simulink model "gm_FCS_MPC_3Phase_SPMSM_TEST1"  (R2022a)
settings: Solver=ode23t  StartTime=0.0  StopTime=0.2  RelTol=1e-3  AbsTol=1e-3  EnableMultiTasking=on
undefined symbols (not defined in the file or in its folder): f_c, Ld, Lq, np, psiPM, R, T_50MHz, u_dc
libraries: dspsigops x31, hdlmdlgenlib x28, ee_lib x22, nesl_utility x22, fl_lib x21, simulink x7
(part 3 of 5)

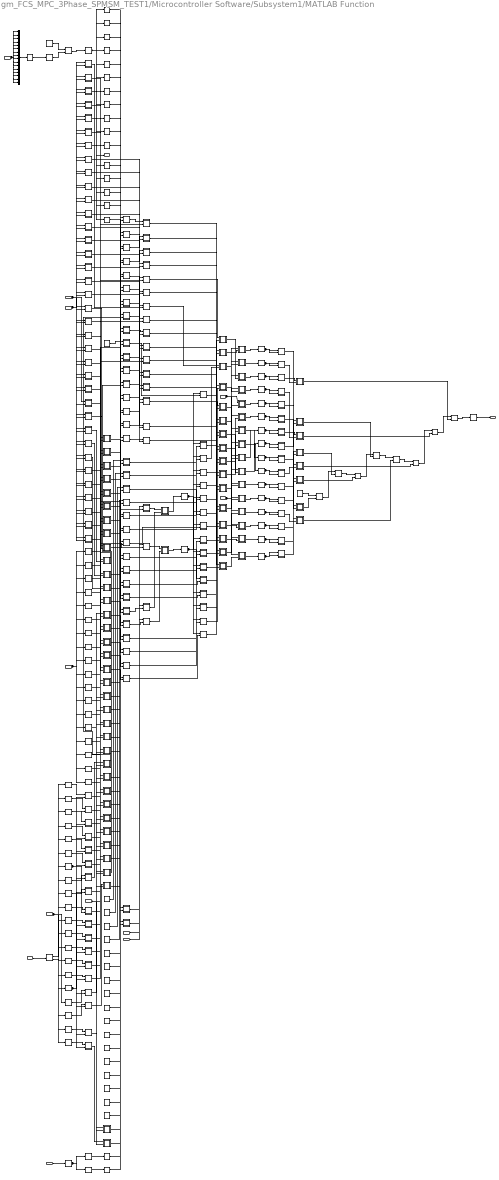
== system gm_FCS_MPC_3Phase_SPMSM_TEST1/Microcontroller Software/Subsystem1/MATLAB Function ==
  u_dc_link : Inport  OutDataTypeStr=single  PortDimensions=1  SampleTime=1e-10
  i_ph_ctrl_alpha : Inport  Port=2  OutDataTypeStr=single  PortDimensions=1  SampleTime=1e-10
  i_ph_ctrl_beta : Inport  Port=3  OutDataTypeStr=single  PortDimensions=1  SampleTime=1e-10
  omega_el : Inport  Port=4  OutDataTypeStr=single  PortDimensions=1  SampleTime=1e-10
  theta_el : Inport  Port=5  OutDataTypeStr=single  PortDimensions=1  SampleTime=1e-10
  Rs : Inport  Port=6  OutDataTypeStr=single  PortDimensions=1  SampleTime=1e-10
  reciprocal_Ls : Inport  Port=7  OutDataTypeStr=single  PortDimensions=1  SampleTime=1e-10
  psiPM : Inport  Port=8  OutDataTypeStr=single  PortDimensions=1  SampleTime=1e-10
  ialpha_ref : Inport  Port=9  OutDataTypeStr=single  PortDimensions=1  SampleTime=1e-10
  ibeta_ref : Inport  Port=10  OutDataTypeStr=single  PortDimensions=1  SampleTime=1e-10
  SampleTime : Inport  Port=11  OutDataTypeStr=single  PortDimensions=1  SampleTime=1e-10
  vk : Inport  Port=12  OutDataTypeStr=single  PortDimensions=[2]  SampleTime=1e-10
  Assignment : Assignment  SampleTime=1e-10  IndexOptions=Index vector (dialog)  Indices=double(8)  OutputSizes=double(0)
  Assignment1 : Assignment  SampleTime=1e-10  IndexOptions=Index vector (dialog)  Indices=double(7)  OutputSizes=double(0)
  Assignment2 : Assignment  SampleTime=1e-10  IndexOptions=Index vector (dialog)  Indices=double(6)  OutputSizes=double(0)
  Assignment3 : Assignment  SampleTime=1e-10  IndexOptions=Index vector (dialog)  Indices=double(5)  OutputSizes=double(0)
  Assignment4 : Assignment  SampleTime=1e-10  IndexOptions=Index vector (dialog)  Indices=double(4)  OutputSizes=double(0)
  Assignment5 : Assignment  SampleTime=1e-10  IndexOptions=Index vector (dialog)  Indices=double(3)  OutputSizes=double(0)
  Assignment6 : Assignment  SampleTime=1e-10  IndexOptions=Index vector (dialog)  Indices=double(2)  OutputSizes=double(0)
  Assignment7 : Assignment  SampleTime=1e-10  IndexOptions=Index vector (dialog)  Indices=double(1)  OutputSizes=double(0)
  Reshape : Reshape
  Reshape1 : Reshape  OutputDimensionality=Column vector (2-D)
  Selector : Selector  NumberOfDimensions=2  SampleTime=1e-10  IndexOptions=Index vector (dialog),Index vector (dialog)  Indices=double(2),double(8)  OutputSizes=double(0),double(0)
  Selector1 : Selector  NumberOfDimensions=2  SampleTime=1e-10  IndexOptions=Index vector (dialog),Index vector (dialog)  Indices=double(1),double(8)  OutputSizes=double(0),double(0)
  Selector10 : Selector  NumberOfDimensions=2  SampleTime=1e-10  IndexOptions=Index vector (dialog),Index vector (dialog)  Indices=double(2),double(4)  OutputSizes=double(0),double(0)
  Selector11 : Selector  NumberOfDimensions=2  SampleTime=1e-10  IndexOptions=Index vector (dialog),Index vector (dialog)  Indices=double(1),double(4)  OutputSizes=double(0),double(0)
  Selector12 : Selector  NumberOfDimensions=2  SampleTime=1e-10  IndexOptions=Index vector (dialog),Index vector (dialog)  Indices=double(2),double(3)  OutputSizes=double(0),double(0)
  Selector13 : Selector  NumberOfDimensions=2  SampleTime=1e-10  IndexOptions=Index vector (dialog),Index vector (dialog)  Indices=double(1),double(3)  OutputSizes=double(0),double(0)
  Selector14 : Selector  NumberOfDimensions=2  SampleTime=1e-10  IndexOptions=Index vector (dialog),Index vector (dialog)  Indices=double(2),double(2)  OutputSizes=double(0),double(0)
  Selector15 : Selector  NumberOfDimensions=2  SampleTime=1e-10  IndexOptions=Index vector (dialog),Index vector (dialog)  Indices=double(1),double(2)  OutputSizes=double(0),double(0)
  Selector16 : Selector  NumberOfDimensions=2  SampleTime=1e-10  IndexOptions=Index vector (dialog),Index vector (dialog)  Indices=double(2),double(1)  OutputSizes=double(0),double(0)
  Selector17 : Selector  NumberOfDimensions=2  SampleTime=1e-10  IndexOptions=Index vector (dialog),Index vector (dialog)  Indices=double(1),double(1)  OutputSizes=double(0),double(0)
  Selector2 : Selector  NumberOfDimensions=2  SampleTime=1e-10  IndexOptions=Index vector (dialog),Index vector (dialog)  Indices=double(2),double(7)  OutputSizes=double(0),double(0)
  Selector3 : Selector  NumberOfDimensions=2  SampleTime=1e-10  IndexOptions=Index vector (dialog),Index vector (dialog)  Indices=double(1),double(7)  OutputSizes=double(0),double(0)
  Selector4 : Selector  SampleTime=1e-10  IndexOptions=Index vector (dialog)  Indices=double(2)  OutputSizes=double(0)
  Selector5 : Selector  SampleTime=1e-10  IndexOptions=Index vector (dialog)  Indices=double(1)  OutputSizes=double(0)
  Selector6 : Selector  NumberOfDimensions=2  SampleTime=1e-10  IndexOptions=Index vector (dialog),Index vector (dialog)  Indices=double(2),double(6)  OutputSizes=double(0),double(0)
  Selector7 : Selector  NumberOfDimensions=2  SampleTime=1e-10  IndexOptions=Index vector (dialog),Index vector (dialog)  Indices=double(1),double(6)  OutputSizes=double(0),double(0)
  Selector8 : Selector  NumberOfDimensions=2  SampleTime=1e-10  IndexOptions=Index vector (dialog),Index vector (dialog)  Indices=double(2),double(5)  OutputSizes=double(0),double(0)
  Selector9 : Selector  NumberOfDimensions=2  SampleTime=1e-10  IndexOptions=Index vector (dialog),Index vector (dialog)  Indices=double(1),double(5)  OutputSizes=double(0),double(0)
  adder : Subsystem
      mask Display: disp('NFP\nadd');
  adder1 : Subsystem
      mask Display: disp('NFP\nadd');
  adder10 : Subsystem
      mask Display: disp('NFP\nadd');
  adder11 : Subsystem
      mask Display: disp('NFP\nadd');
  adder12 : Subsystem
      mask Display: disp('NFP\nadd');
  adder13 : Subsystem
      mask Display: disp('NFP\nadd');
  adder14 : Subsystem
      mask Display: disp('NFP\nadd');
  adder15 : Subsystem
      mask Display: disp('NFP\nadd');
  adder16 : Subsystem
      mask Display: disp('NFP\nadd');
  adder17 : Subsystem
      mask Display: disp('NFP\nadd');
  adder18 : Subsystem
      mask Display: disp('NFP\nadd');
  adder19 : Subsystem
      mask Display: disp('NFP\nadd');
  adder2 : Subsystem
      mask Display: disp('NFP\nadd');
  adder20 : Subsystem
      mask Display: disp('NFP\nadd');
  adder21 : Subsystem
      mask Display: disp('NFP\nadd');
  adder22 : Subsystem
      mask Display: disp('NFP\nadd');
  adder23 : Subsystem
      mask Display: disp('NFP\nadd');
  adder24 : Subsystem
      mask Display: disp('NFP\nadd');
  adder25 : Subsystem
      mask Display: disp('NFP\nadd');
  adder26 : Subsystem
      mask Display: disp('NFP\nadd');
  adder27 : Subsystem
      mask Display: disp('NFP\nadd');
  adder28 : Subsystem
      mask Display: disp('NFP\nadd');
  adder29 : Subsystem
      mask Display: disp('NFP\nadd');
  adder3 : Subsystem
      mask Display: disp('NFP\nadd');
  adder30 : Subsystem
      mask Display: disp('NFP\nadd');
  adder31 : Subsystem
      mask Display: disp('NFP\nadd');
  adder32 : Subsystem
      mask Display: disp('NFP\nadd');
  adder33 : Subsystem
      mask Display: disp('NFP\nadd');
  adder34 : Subsystem
      mask Display: disp('NFP\nadd');
  adder4 : Subsystem
      mask Display: disp('NFP\nadd');
  adder5 : Subsystem
      mask Display: disp('NFP\nadd');
  adder6 : Subsystem
      mask Display: disp('NFP\nadd');
  adder7 : Subsystem
      mask Display: disp('NFP\nadd');
  adder8 : Subsystem
      mask Display: disp('NFP\nadd');
  adder9 : Subsystem
      mask Display: disp('NFP\nadd');
  adder_outbuff : hdlmdlgenlib/Buffer
      settings: SourceProductBaseCode=SL
  adder_outbuff1 : hdlmdlgenlib/Buffer
      settings: SourceProductBaseCode=SL
  concatenate : Concatenate  NumInputs=16
  const{,1..3,5..18} (18 alike) : Constant  Value=single(1)  VectorParams1D=off  OutDataTypeStr=single  SampleTime=1e-10
  const4 : Constant  Value="repmat(single(0),[8  1])"  VectorParams1D=off  OutDataTypeStr=single  SampleTime=1e-10
  cos_to_sincos : Subsystem
      mask Display: disp('NFP\ntrig2');
  cos_to_sincos_out1_buff : hdlmdlgenlib/Buffer
      settings: SourceProductBaseCode=SL
  cos_to_sincos_out2_buff : hdlmdlgenlib/Buffer
      settings: SourceProductBaseCode=SL
  delayMatch{,1..37} (38 alike) : Delay  DelayLength=double(1)  InitialCondition=0  SampleTime=1e-10
  gain : Reshape  OutputDimensionality=Customize  OutputDimensions=[2,8]
  gain1 : Subsystem
      mask Display: disp('NFP\nmul');
  gain_const : Constant  Value=single([0 0 0.6666666865348816 0 0.3333333432674408 0.5774 -0.3333333432674408 0.5774 -0.6666666865348816 0 -0.3333333432674408 -0.5774 0.3333333432674408 -0.5774 0 0]).'  OutDataTypeStr=single  SampleTime=1e-10
  multiplier : Subsystem
      mask Display: disp('NFP\nmul');
  multiplier1 : Subsystem
      mask Display: disp('NFP\nmul');
  multiplier10 : Subsystem
      mask Display: disp('NFP\nmul');
  multiplier100 : Subsystem
      mask Display: disp('NFP\nmul');
  multiplier101 : Subsystem
      mask Display: disp('NFP\nmul');
  multiplier102 : Subsystem
      mask Display: disp('NFP\nmul');
  multiplier103 : Subsystem
      mask Display: disp('NFP\nmul');
  multiplier104 : Subsystem
      mask Display: disp('NFP\nmul');
  multiplier105 : Subsystem
      mask Display: disp('NFP\nmul');
  multiplier106 : Subsystem
      mask Display: disp('NFP\nmul');
  multiplier107 : Subsystem
      mask Display: disp('NFP\nmul');
  multiplier108 : Subsystem
      mask Display: disp('NFP\nmul');
  multiplier109 : Subsystem
      mask Display: disp('NFP\nmul');
  multiplier11 : Subsystem
      mask Display: disp('NFP\nmul');
  multiplier110 : Subsystem
      mask Display: disp('NFP\nmul');
  multiplier111 : Subsystem
      mask Display: disp('NFP\nmul');
  multiplier112 : Subsystem
      mask Display: disp('NFP\nmul');
  multiplier113 : Subsystem
      mask Display: disp('NFP\nmul');
  multiplier114 : Subsystem
      mask Display: disp('NFP\nmul');
  multiplier115 : Subsystem
      mask Display: disp('NFP\nmul');
  multiplier116 : Subsystem
      mask Display: disp('NFP\nmul');
  multiplier117 : Subsystem
      mask Display: disp('NFP\nmul');
  multiplier118 : Subsystem
      mask Display: disp('NFP\nmul');
  multiplier119 : Subsystem
      mask Display: disp('NFP\nmul');
  multiplier12 : Subsystem
      mask Display: disp('NFP\nmul');
  multiplier120 : Subsystem
      mask Display: disp('NFP\nmul');
  multiplier121 : Subsystem
      mask Display: disp('NFP\nmul');
  multiplier122 : Subsystem
      mask Display: disp('NFP\nmul');
  multiplier123 : Subsystem
      mask Display: disp('NFP\nmul');
  multiplier124 : Subsystem
      mask Display: disp('NFP\nmul');
  multiplier125 : Subsystem
      mask Display: disp('NFP\nmul');
  multiplier13 : Subsystem
      mask Display: disp('NFP\nmul');
  multiplier14 : Subsystem
      mask Display: disp('NFP\nmul');
  multiplier15 : Subsystem
      mask Display: disp('NFP\nmul');
  multiplier16 : Subsystem
      mask Display: disp('NFP\nmul');
  multiplier17 : Subsystem
      mask Display: disp('NFP\nmul');
  multiplier18 : Subsystem
      mask Display: disp('NFP\nmul');
  multiplier19 : Subsystem
      mask Display: disp('NFP\nmul');
  multiplier2 : Subsystem
      mask Display: disp('NFP\nmul');
  multiplier20 : Subsystem
      mask Display: disp('NFP\nmul');
  multiplier21 : Subsystem
      mask Display: disp('NFP\nmul');
  multiplier22 : Subsystem
      mask Display: disp('NFP\nmul');
  multiplier23 : Subsystem
      mask Display: disp('NFP\nmul');
  multiplier24 : Subsystem
      mask Display: disp('NFP\nmul');
  multiplier25 : Subsystem
      mask Display: disp('NFP\nmul');
  multiplier26 : Subsystem
      mask Display: disp('NFP\nmul');
  multiplier27 : Subsystem
      mask Display: disp('NFP\nmul');
  multiplier28 : Subsystem
      mask Display: disp('NFP\nmul');
  multiplier29 : Subsystem
      mask Display: disp('NFP\nmul');
  multiplier3 : Subsystem
      mask Display: disp('NFP\nmul');
  multiplier30 : Subsystem
      mask Display: disp('NFP\nmul');
  multiplier31 : Subsystem
      mask Display: disp('NFP\nmul');
  multiplier32 : Subsystem
      mask Display: disp('NFP\nmul');
  multiplier33 : Subsystem
      mask Display: disp('NFP\nmul');
  multiplier34 : Subsystem
      mask Display: disp('NFP\nmul');
  multiplier35 : Subsystem
      mask Display: disp('NFP\nmul');
  multiplier36 : Subsystem
      mask Display: disp('NFP\nmul');
  multiplier37 : Subsystem
      mask Display: disp('NFP\nmul');
  multiplier38 : Subsystem
      mask Display: disp('NFP\nmul');
  multiplier39 : Subsystem
      mask Display: disp('NFP\nmul');
  multiplier4 : Subsystem
      mask Display: disp('NFP\nmul');
  multiplier40 : Subsystem
      mask Display: disp('NFP\nmul');
  multiplier41 : Subsystem
      mask Display: disp('NFP\nmul');
  multiplier42 : Subsystem
      mask Display: disp('NFP\nmul');
  multiplier43 : Subsystem
      mask Display: disp('NFP\nmul');
  multiplier44 : Subsystem
      mask Display: disp('NFP\nmul');
  multiplier45 : Subsystem
      mask Display: disp('NFP\nmul');
  multiplier46 : Subsystem
      mask Display: disp('NFP\nmul');
  multiplier47 : Subsystem
      mask Display: disp('NFP\nmul');
  multiplier48 : Subsystem
      mask Display: disp('NFP\nmul');
  multiplier49 : Subsystem
      mask Display: disp('NFP\nmul');
  multiplier5 : Subsystem
      mask Display: disp('NFP\nmul');
  multiplier50 : Subsystem
      mask Display: disp('NFP\nmul');
  multiplier51 : Subsystem
      mask Display: disp('NFP\nmul');
  multiplier52 : Subsystem
      mask Display: disp('NFP\nmul');
  multiplier53 : Subsystem
      mask Display: disp('NFP\nmul');
  multiplier54 : Subsystem
      mask Display: disp('NFP\nmul');
  multiplier55 : Subsystem
      mask Display: disp('NFP\nmul');
  multiplier56 : Subsystem
      mask Display: disp('NFP\nmul');
  multiplier57 : Subsystem
      mask Display: disp('NFP\nmul');
  multiplier58 : Subsystem
      mask Display: disp('NFP\nmul');
  multiplier59 : Subsystem
      mask Display: disp('NFP\nmul');
  multiplier6 : Subsystem
      mask Display: disp('NFP\nmul');
  multiplier60 : Subsystem
      mask Display: disp('NFP\nmul');
  multiplier61 : Subsystem
      mask Display: disp('NFP\nmul');
  multiplier62 : Subsystem
      mask Display: disp('NFP\nmul');
  multiplier63 : Subsystem
      mask Display: disp('NFP\nmul');
  multiplier64 : Subsystem
      mask Display: disp('NFP\nmul');
  multiplier65 : Subsystem
      mask Display: disp('NFP\nmul');
  multiplier66 : Subsystem
      mask Display: disp('NFP\nmul');
  multiplier67 : Subsystem
      mask Display: disp('NFP\nmul');
  multiplier68 : Subsystem
      mask Display: disp('NFP\nmul');
  multiplier69 : Subsystem
      mask Display: disp('NFP\nmul');
  multiplier7 : Subsystem
      mask Display: disp('NFP\nmul');
  multiplier70 : Subsystem
      mask Display: disp('NFP\nmul');
  multiplier71 : Subsystem
      mask Display: disp('NFP\nmul');
  multiplier72 : Subsystem
      mask Display: disp('NFP\nmul');
  multiplier73 : Subsystem
      mask Display: disp('NFP\nmul');
  multiplier74 : Subsystem
      mask Display: disp('NFP\nmul');
  multiplier75 : Subsystem
      mask Display: disp('NFP\nmul');
  multiplier76 : Subsystem
      mask Display: disp('NFP\nmul');
  multiplier77 : Subsystem
      mask Display: disp('NFP\nmul');
  multiplier78 : Subsystem
      mask Display: disp('NFP\nmul');
  multiplier79 : Subsystem
      mask Display: disp('NFP\nmul');
  multiplier8 : Subsystem
      mask Display: disp('NFP\nmul');
  multiplier80 : Subsystem
      mask Display: disp('NFP\nmul');
  multiplier81 : Subsystem
      mask Display: disp('NFP\nmul');
  multiplier82 : Subsystem
      mask Display: disp('NFP\nmul');
  multiplier83 : Subsystem
      mask Display: disp('NFP\nmul');
  multiplier84 : Subsystem
      mask Display: disp('NFP\nmul');
  multiplier85 : Subsystem
      mask Display: disp('NFP\nmul');
  multiplier86 : Subsystem
      mask Display: disp('NFP\nmul');
  multiplier87 : Subsystem
      mask Display: disp('NFP\nmul');
  multiplier88 : Subsystem
      mask Display: disp('NFP\nmul');
  multiplier89 : Subsystem
      mask Display: disp('NFP\nmul');
  multiplier9 : Subsystem
      mask Display: disp('NFP\nmul');
  multiplier90 : Subsystem
      mask Display: disp('NFP\nmul');
  multiplier91 : Subsystem
      mask Display: disp('NFP\nmul');
  multiplier92 : Subsystem
      mask Display: disp('NFP\nmul');
  multiplier93 : Subsystem
      mask Display: disp('NFP\nmul');
  multiplier94 : Subsystem
      mask Display: disp('NFP\nmul');
  multiplier95 : Subsystem
      mask Display: disp('NFP\nmul');
  multiplier96 : Subsystem
      mask Display: disp('NFP\nmul');
  multiplier97 : Subsystem
      mask Display: disp('NFP\nmul');
  multiplier98 : Subsystem
      mask Display: disp('NFP\nmul');
  multiplier99 : Subsystem
      mask Display: disp('NFP\nmul');
  square : Subsystem
      mask Display: disp('NFP\nmul');
  square1 : Subsystem
      mask Display: disp('NFP\nmul');
  square10 : Subsystem
      mask Display: disp('NFP\nmul');
  square11 : Subsystem
      mask Display: disp('NFP\nmul');
  square12 : Subsystem
      mask Display: disp('NFP\nmul');
  square13 : Subsystem
      mask Display: disp('NFP\nmul');
  square14 : Subsystem
      mask Display: disp('NFP\nmul');
  square15 : Subsystem
      mask Display: disp('NFP\nmul');
  square2 : Subsystem
      mask Display: disp('NFP\nmul');
  square3 : Subsystem
      mask Display: disp('NFP\nmul');
  square4 : Subsystem
      mask Display: disp('NFP\nmul');
  square5 : Subsystem
      mask Display: disp('NFP\nmul');
  square6 : Subsystem
      mask Display: disp('NFP\nmul');
  square7 : Subsystem
      mask Display: disp('NFP\nmul');
  square8 : Subsystem
      mask Display: disp('NFP\nmul');
  square9 : Subsystem
      mask Display: disp('NFP\nmul');
  subtract : Subsystem
      mask Display: disp('NFP\nadd');
  subtract1 : Subsystem
      mask Display: disp('NFP\nadd');
  subtract10 : Subsystem
      mask Display: disp('NFP\nadd');
  subtract11 : Subsystem
      mask Display: disp('NFP\nadd');
  subtract12 : Subsystem
      mask Display: disp('NFP\nadd');
  subtract13 : Subsystem
      mask Display: disp('NFP\nadd');
  subtract14 : Subsystem
      mask Display: disp('NFP\nadd');
  subtract15 : Subsystem
      mask Display: disp('NFP\nadd');
  subtract16 : Subsystem
      mask Display: disp('NFP\nadd');
  subtract17 : Subsystem
      mask Display: disp('NFP\nadd');
  subtract18 : Subsystem
      mask Display: disp('NFP\nadd');
  subtract19 : Subsystem
      mask Display: disp('NFP\nadd');
  subtract2 : Subsystem
      mask Display: disp('NFP\nadd');
  subtract20 : Subsystem
      mask Display: disp('NFP\nadd');
  subtract21 : Subsystem
      mask Display: disp('NFP\nadd');
  subtract22 : Subsystem
      mask Display: disp('NFP\nadd');
  subtract23 : Subsystem
      mask Display: disp('NFP\nadd');
  subtract24 : Subsystem
      mask Display: disp('NFP\nadd');
  subtract25 : Subsystem
      mask Display: disp('NFP\nadd');
  subtract26 : Subsystem
      mask Display: disp('NFP\nadd');
  subtract27 : Subsystem
      mask Display: disp('NFP\nadd');
  subtract28 : Subsystem
      mask Display: disp('NFP\nadd');
  subtract29 : Subsystem
      mask Display: disp('NFP\nadd');
  subtract3 : Subsystem
      mask Display: disp('NFP\nadd');
  subtract30 : Subsystem
      mask Display: disp('NFP\nadd');
  subtract31 : Subsystem
      mask Display: disp('NFP\nadd');
  subtract32 : Subsystem
      mask Display: disp('NFP\nadd');
  subtract33 : Subsystem
      mask Display: disp('NFP\nadd');
  subtract34 : Subsystem
      mask Display: disp('NFP\nadd');
  subtract35 : Subsystem
      mask Display: disp('NFP\nadd');
  subtract36 : Subsystem
      mask Display: disp('NFP\nadd');
  subtract37 : Subsystem
      mask Display: disp('NFP\nadd');
  subtract38 : Subsystem
      mask Display: disp('NFP\nadd');
  subtract39 : Subsystem
      mask Display: disp('NFP\nadd');
  subtract4 : Subsystem
      mask Display: disp('NFP\nadd');
  subtract40 : Subsystem
      mask Display: disp('NFP\nadd');
  subtract41 : Subsystem
      mask Display: disp('NFP\nadd');
  subtract42 : Subsystem
      mask Display: disp('NFP\nadd');
  subtract5 : Subsystem
      mask Display: disp('NFP\nadd');
  subtract6 : Subsystem
      mask Display: disp('NFP\nadd');
  subtract7 : Subsystem
      mask Display: disp('NFP\nadd');
  subtract8 : Subsystem
      mask Display: disp('NFP\nadd');
  subtract9 : Subsystem
      mask Display: disp('NFP\nadd');
  subtract_outbuff{,1..15} (16 alike) : hdlmdlgenlib/Buffer
      settings: SourceProductBaseCode=SL
  t : Reshape  OutputDimensionality=Column vector (2-D)
  t1 : Reshape  OutputDimensionality=Customize  OutputDimensions=[2,8]
  J : Outport  SampleTime=1e-10  VectorParamsAs1DForOutWhenUnconnected=off
  v : Outport  Port=2  SampleTime=1e-10
  wires:
  Reshape/1 -> J/1
  t1/1 -> Selector17/1, Selector16/1, Selector15/1, Selector14/1, Selector13/1, Selector12/1, Selector11/1, Selector10/1, Selector9/1, Selector8/1, Selector7/1, Selector6/1, Selector3/1, Selector2/1, Selector1/1, Selector/1, v/1
  Assignment/1 -> Reshape/1
  gain/1 -> t/1
  Assignment1/1 -> Assignment/1
  concatenate/1 -> gain/1
  Assignment2/1 -> Assignment1/1
  subtract_outbuff/1 -> square/2(In2), square/1(In1)
  subtract_outbuff1/1 -> square1/2(In2), square1/1(In1)
  Assignment3/1 -> Assignment2/1
  subtract_outbuff2/1 -> square2/2(In2), square2/1(In1)
  subtract_outbuff3/1 -> square3/2(In2), square3/1(In1)
  Assignment4/1 -> Assignment3/1
  subtract_outbuff4/1 -> square4/2(In2), square4/1(In1)
  subtract_outbuff5/1 -> square5/2(In2), square5/1(In1)
  Assignment5/1 -> Assignment4/1
  adder_outbuff/1 -> multiplier100/1(In1), multiplier86/1(In1), multiplier72/1(In1), multiplier54/1(In1), multiplier36/1(In1), multiplier20/1(In1), multiplier6/1(In1), multiplier/1(In1)
  adder_outbuff1/1 -> multiplier102/1(In1), multiplier88/1(In1), multiplier74/1(In1), multiplier56/1(In1), multiplier38/1(In1), multiplier22/1(In1), multiplier8/1(In1), multiplier2/1(In1)
  subtract_outbuff6/1 -> square6/2(In2), square6/1(In1)
  subtract_outbuff7/1 -> square7/2(In2), square7/1(In1)
  Assignment6/1 -> Assignment5/1
  const/1 -> subtract6/1(In1)
  const1/1 -> subtract8/1(In1)
  subtract_outbuff8/1 -> square8/2(In2), square8/1(In1)
  subtract_outbuff9/1 -> square9/2(In2), square9/1(In1)
  Assignment7/1 -> Assignment6/1
  const2/1 -> subtract11/1(In1)
  const3/1 -> subtract13/1(In1)
  subtract_outbuff10/1 -> square10/2(In2), square10/1(In1)
  subtract_outbuff11/1 -> square11/2(In2), square11/1(In1)
  const4/1 -> Assignment7/1
  const5/1 -> subtract16/1(In1)
  cos_to_sincos_out2_buff/1 -> multiplier123/2(In2), multiplier115/2(In2), multiplier105/2(In2), multiplier91/2(In2), multiplier77/2(In2), multiplier63/2(In2), multiplier59/2(In2), multiplier45/2(In2), multiplier26/2(In2)
  const6/1 -> subtract18/1(In1)
  cos_to_sincos_out1_buff/1 -> multiplier125/2(In2), multiplier117/2(In2), multiplier107/2(In2), multiplier93/2(In2), multiplier79/2(In2), multiplier65/2(In2), multiplier61/2(In2), multiplier47/2(In2), multiplier29/2(In2)
  const7/1 -> subtract19/1(In1)
  const8/1 -> subtract21/1(In1)
  subtract_outbuff12/1 -> square12/2(In2), square12/1(In1)
  subtract_outbuff13/1 -> square13/2(In2), square13/1(In1)
  Reshape1/1 -> Selector5/1, Selector4/1
  const9/1 -> subtract24/1(In1)
  const10/1 -> subtract26/1(In1)
  subtract_outbuff14/1 -> square14/2(In2), square14/1(In1)
  subtract_outbuff15/1 -> square15/2(In2), square15/1(In1)
  const11/1 -> subtract29/1(In1)
  const12/1 -> subtract31/1(In1)
  const13/1 -> subtract34/1(In1)
  const14/1 -> subtract36/1(In1)
  const15/1 -> subtract37/1(In1)
  const16/1 -> subtract39/1(In1)
  const17/1 -> subtract40/1(In1)
  const18/1 -> subtract42/1(In1)
  t/1 -> gain1/2(In2)
  gain_const/1 -> gain1/1(In1)
  delayMatch3/1 -> multiplier42/1(In1)
  adder/1(Out1) -> Assignment/2
  square/1(Out1) -> adder/2(In2)
  square1/1(Out1) -> adder/1(In1)
  adder1/1(Out1) -> Assignment1/2
  subtract/1(Out1) -> subtract_outbuff/1
  subtract1/1(Out1) -> subtract_outbuff1/1
  square2/1(Out1) -> adder1/2(In2)
  square3/1(Out1) -> adder1/1(In1)
  adder2/1(Out1) -> Assignment2/2
  adder3/1(Out1) -> subtract/2(In2)
  adder4/1(Out1) -> subtract1/2(In2)
  subtract2/1(Out1) -> subtract_outbuff2/1
  subtract3/1(Out1) -> subtract_outbuff3/1
  square4/1(Out1) -> adder2/2(In2)
  square5/1(Out1) -> adder2/1(In1)
  adder5/1(Out1) -> Assignment3/2
  multiplier/1(Out1) -> adder3/2(In2)
  multiplier1/1(Out1) -> adder3/1(In1)
  multiplier2/1(Out1) -> adder4/2(In2)
  multiplier3/1(Out1) -> adder4/1(In1)
  adder6/1(Out1) -> subtract2/2(In2)
  adder7/1(Out1) -> subtract3/2(In2)
  subtract4/1(Out1) -> subtract_outbuff4/1
  subtract5/1(Out1) -> subtract_outbuff5/1
  square6/1(Out1) -> adder5/2(In2)
  square7/1(Out1) -> adder5/1(In1)
  adder8/1(Out1) -> Assignment4/2
  subtract6/1(Out1) -> multiplier/2(In2)
  adder9/1(Out1) -> adder_outbuff/1
  multiplier4/1(Out1) -> multiplier1/2(In2)
  subtract7/1(Out1) -> multiplier1/1(In1)
  subtract8/1(Out1) -> multiplier2/2(In2)
  adder10/1(Out1) -> adder_outbuff1/1
  multiplier5/1(Out1) -> multiplier3/2(In2)
  adder11/1(Out1) -> multiplier3/1(In1)
  multiplier6/1(Out1) -> adder6/2(In2)
  multiplier7/1(Out1) -> adder6/1(In1)
  multiplier8/1(Out1) -> adder7/2(In2)
  multiplier9/1(Out1) -> adder7/1(In1)
  adder12/1(Out1) -> subtract4/2(In2)
  adder13/1(Out1) -> subtract5/2(In2)
  subtract9/1(Out1) -> subtract_outbuff6/1
  subtract10/1(Out1) -> subtract_outbuff7/1
  square8/1(Out1) -> adder8/2(In2)
  square9/1(Out1) -> adder8/1(In1)
  adder14/1(Out1) -> Assignment5/2
  multiplier10/1(Out1) -> subtract6/2(In2)
  multiplier11/1(Out1) -> adder9/2(In2)
  multiplier12/1(Out1) -> adder9/1(In1)
  multiplier13/1(Out1) -> subtract7/2(In2)
  multiplier14/1(Out1) -> subtract8/2(In2)
  multiplier15/1(Out1) -> adder10/2(In2)
  multiplier16/1(Out1) -> adder10/1(In1)
  multiplier17/1(Out1) -> adder11/2(In2)
  subtract11/1(Out1) -> multiplier6/2(In2)
  multiplier18/1(Out1) -> multiplier7/2(In2)
  subtract12/1(Out1) -> multiplier7/1(In1)
  subtract13/1(Out1) -> multiplier8/2(In2)
  multiplier19/1(Out1) -> multiplier9/2(In2)
  adder15/1(Out1) -> multiplier9/1(In1)
  multiplier20/1(Out1) -> adder12/2(In2)
  multiplier21/1(Out1) -> adder12/1(In1)
  multiplier22/1(Out1) -> adder13/2(In2)
  multiplier23/1(Out1) -> adder13/1(In1)
  adder16/1(Out1) -> subtract9/2(In2)
  adder17/1(Out1) -> subtract10/2(In2)
  subtract14/1(Out1) -> subtract_outbuff8/1
  subtract15/1(Out1) -> subtract_outbuff9/1
  square10/1(Out1) -> adder14/2(In2)
  square11/1(Out1) -> adder14/1(In1)
  adder18/1(Out1) -> Assignment6/2
  multiplier24/1(Out1) -> multiplier10/2(In2)
  subtract16/1(Out1) -> multiplier11/2(In2)
  multiplier25/1(Out1) -> multiplier12/2(In2)
  subtract17/1(Out1) -> multiplier12/1(In1)
  multiplier26/1(Out1) -> multiplier13/1(In1)
  multiplier27/1(Out1) -> multiplier14/2(In2)
  subtract18/1(Out1) -> multiplier15/2(In2)
  multiplier28/1(Out1) -> multiplier16/2(In2)
  adder19/1(Out1) -> multiplier16/1(In1)
  multiplier29/1(Out1) -> multiplier17/1(In1)
  multiplier30/1(Out1) -> subtract11/2(In2)
  multiplier31/1(Out1) -> subtract12/2(In2)
  multiplier32/1(Out1) -> subtract13/2(In2)
  multiplier33/1(Out1) -> adder15/2(In2)
  subtract19/1(Out1) -> multiplier20/2(In2)
  multiplier34/1(Out1) -> multiplier21/2(In2)
  subtract20/1(Out1) -> multiplier21/1(In1)
  subtract21/1(Out1) -> multiplier22/2(In2)
  multiplier35/1(Out1) -> multiplier23/2(In2)
  adder20/1(Out1) -> multiplier23/1(In1)
  multiplier36/1(Out1) -> adder16/2(In2)
  multiplier37/1(Out1) -> adder16/1(In1)
  multiplier38/1(Out1) -> adder17/2(In2)
  multiplier39/1(Out1) -> adder17/1(In1)
  adder21/1(Out1) -> subtract14/2(In2)
  adder22/1(Out1) -> subtract15/2(In2)
  subtract22/1(Out1) -> subtract_outbuff10/1
  subtract23/1(Out1) -> subtract_outbuff11/1
  square12/1(Out1) -> adder18/2(In2)
  square13/1(Out1) -> adder18/1(In1)
  adder23/1(Out1) -> Assignment7/2
  multiplier40/1(Out1) -> subtract16/2(In2)
  multiplier41/1(Out1) -> subtract17/2(In2)
  multiplier42/1(Out1) -> subtract18/2(In2)
  multiplier43/1(Out1) -> adder19/2(In2)
  multiplier44/1(Out1) -> multiplier30/2(In2)
  multiplier45/1(Out1) -> multiplier31/1(In1)
  multiplier46/1(Out1) -> multiplier32/2(In2)
  multiplier47/1(Out1) -> multiplier33/1(In1)
  multiplier48/1(Out1) -> subtract19/2(In2)
  multiplier49/1(Out1) -> subtract20/2(In2)
  multiplier50/1(Out1) -> subtract21/2(In2)
  multiplier51/1(Out1) -> adder20/2(In2)
  subtract24/1(Out1) -> multiplier36/2(In2)
  multiplier52/1(Out1) -> multiplier37/2(In2)
  subtract25/1(Out1) -> multiplier37/1(In1)
  subtract26/1(Out1) -> multiplier38/2(In2)
  multiplier53/1(Out1) -> multiplier39/2(In2)
  adder24/1(Out1) -> multiplier39/1(In1)
  multiplier54/1(Out1) -> adder21/2(In2)
  multiplier55/1(Out1) -> adder21/1(In1)
  multiplier56/1(Out1) -> adder22/2(In2)
  multiplier57/1(Out1) -> adder22/1(In1)
  adder25/1(Out1) -> subtract22/2(In2)
  adder26/1(Out1) -> subtract23/2(In2)
  subtract27/1(Out1) -> subtract_outbuff12/1
  subtract28/1(Out1) -> subtract_outbuff13/1
  square14/1(Out1) -> adder23/2(In2)
  square15/1(Out1) -> adder23/1(In1)
  multiplier58/1(Out1) -> multiplier40/2(In2)
  multiplier59/1(Out1) -> multiplier41/1(In1)
  multiplier60/1(Out1) -> multiplier42/2(In2)
  multiplier61/1(Out1) -> multiplier43/1(In1)
  multiplier62/1(Out1) -> multiplier48/2(In2)
  multiplier63/1(Out1) -> multiplier49/1(In1)
  multiplier64/1(Out1) -> multiplier50/2(In2)
  multiplier65/1(Out1) -> multiplier51/1(In1)
  multiplier66/1(Out1) -> subtract24/2(In2)
  multiplier67/1(Out1) -> subtract25/2(In2)
  multiplier68/1(Out1) -> subtract26/2(In2)
  multiplier69/1(Out1) -> adder24/2(In2)
  subtract29/1(Out1) -> multiplier54/2(In2)
  multiplier70/1(Out1) -> multiplier55/2(In2)
  subtract30/1(Out1) -> multiplier55/1(In1)
  subtract31/1(Out1) -> multiplier56/2(In2)
  multiplier71/1(Out1) -> multiplier57/2(In2)
  adder27/1(Out1) -> multiplier57/1(In1)
  multiplier72/1(Out1) -> adder25/2(In2)
  multiplier73/1(Out1) -> adder25/1(In1)
  multiplier74/1(Out1) -> adder26/2(In2)
  multiplier75/1(Out1) -> adder26/1(In1)
  adder28/1(Out1) -> subtract27/2(In2)
  adder29/1(Out1) -> subtract28/2(In2)
  subtract32/1(Out1) -> subtract_outbuff14/1
  subtract33/1(Out1) -> subtract_outbuff15/1
  multiplier76/1(Out1) -> multiplier66/2(In2)
  multiplier77/1(Out1) -> multiplier67/1(In1)
  multiplier78/1(Out1) -> multiplier68/2(In2)
  multiplier79/1(Out1) -> multiplier69/1(In1)
  multiplier80/1(Out1) -> subtract29/2(In2)
  multiplier81/1(Out1) -> subtract30/2(In2)
  multiplier82/1(Out1) -> subtract31/2(In2)
  multiplier83/1(Out1) -> adder27/2(In2)
  subtract34/1(Out1) -> multiplier72/2(In2)
  multiplier84/1(Out1) -> multiplier73/2(In2)
  subtract35/1(Out1) -> multiplier73/1(In1)
  subtract36/1(Out1) -> multiplier74/2(In2)
  multiplier85/1(Out1) -> multiplier75/2(In2)
  adder30/1(Out1) -> multiplier75/1(In1)
  multiplier86/1(Out1) -> adder28/2(In2)
  multiplier87/1(Out1) -> adder28/1(In1)
  multiplier88/1(Out1) -> adder29/2(In2)
  multiplier89/1(Out1) -> adder29/1(In1)
  adder31/1(Out1) -> subtract32/2(In2)
  adder32/1(Out1) -> subtract33/2(In2)
  multiplier90/1(Out1) -> multiplier80/2(In2)
  multiplier91/1(Out1) -> multiplier81/1(In1)
  multiplier92/1(Out1) -> multiplier82/2(In2)
  multiplier93/1(Out1) -> multiplier83/1(In1)
  multiplier94/1(Out1) -> subtract34/2(In2)
  multiplier95/1(Out1) -> subtract35/2(In2)
  multiplier96/1(Out1) -> subtract36/2(In2)
  multiplier97/1(Out1) -> adder30/2(In2)
  subtract37/1(Out1) -> multiplier86/2(In2)
  multiplier98/1(Out1) -> multiplier87/2(In2)
  subtract38/1(Out1) -> multiplier87/1(In1)
  subtract39/1(Out1) -> multiplier88/2(In2)
  multiplier99/1(Out1) -> multiplier89/2(In2)
  adder33/1(Out1) -> multiplier89/1(In1)
  multiplier100/1(Out1) -> adder31/2(In2)
  multiplier101/1(Out1) -> adder31/1(In1)
  multiplier102/1(Out1) -> adder32/2(In2)
  multiplier103/1(Out1) -> adder32/1(In1)
  multiplier104/1(Out1) -> multiplier94/2(In2)
  multiplier105/1(Out1) -> multiplier95/1(In1)
  multiplier106/1(Out1) -> multiplier96/2(In2)
  multiplier107/1(Out1) -> multiplier97/1(In1)
  multiplier108/1(Out1) -> subtract37/2(In2)
  multiplier109/1(Out1) -> subtract38/2(In2)
  multiplier110/1(Out1) -> subtract39/2(In2)
  multiplier111/1(Out1) -> adder33/2(In2)
  subtract40/1(Out1) -> multiplier100/2(In2)
  multiplier112/1(Out1) -> multiplier101/2(In2)
  subtract41/1(Out1) -> multiplier101/1(In1)
  subtract42/1(Out1) -> multiplier102/2(In2)
  multiplier113/1(Out1) -> multiplier103/2(In2)
  adder34/1(Out1) -> multiplier103/1(In1)
  multiplier114/1(Out1) -> multiplier108/2(In2)
  multiplier115/1(Out1) -> multiplier109/1(In1)
  multiplier116/1(Out1) -> multiplier110/2(In2)
  multiplier117/1(Out1) -> multiplier111/1(In1)
  multiplier118/1(Out1) -> subtract40/2(In2)
  multiplier119/1(Out1) -> subtract41/2(In2)
  multiplier120/1(Out1) -> subtract42/2(In2)
  multiplier121/1(Out1) -> adder34/2(In2)
  multiplier122/1(Out1) -> multiplier118/2(In2)
  multiplier123/1(Out1) -> multiplier119/1(In1)
  multiplier124/1(Out1) -> multiplier120/2(In2)
  multiplier125/1(Out1) -> multiplier121/1(In1)
  cos_to_sincos/1(Out1) -> cos_to_sincos_out1_buff/1
  cos_to_sincos/2(Out2) -> cos_to_sincos_out2_buff/1
  gain1/1(Out1) -> t1/1
  Selector5/1 -> delayMatch2/1
  delayMatch4/1 -> multiplier120/1(In1)
  delayMatch8/1 -> multiplier40/1(In1)
  Selector17/1 -> adder34/1(In1)
  Selector4/1 -> delayMatch7/1
  delayMatch9/1 -> multiplier118/1(In1)
  delayMatch11/1 -> multiplier110/1(In1)
  Selector16/1 -> subtract41/1(In1)
  delayMatch13/1 -> multiplier108/1(In1)
  Selector15/1 -> adder33/1(In1)
  delayMatch15/1 -> multiplier96/1(In1)
  Selector14/1 -> subtract38/1(In1)
  delayMatch17/1 -> multiplier94/1(In1)
  Selector13/1 -> adder30/1(In1)
  delayMatch19/1 -> multiplier82/1(In1)
  Selector12/1 -> subtract35/1(In1)
  delayMatch21/1 -> multiplier80/1(In1)
  Selector11/1 -> adder27/1(In1)
  delayMatch23/1 -> multiplier68/1(In1)
  Selector10/1 -> subtract30/1(In1)
  delayMatch25/1 -> multiplier66/1(In1)
  Selector9/1 -> adder24/1(In1)
  delayMatch27/1 -> multiplier50/1(In1)
  Selector8/1 -> subtract25/1(In1)
  delayMatch29/1 -> multiplier48/1(In1)
  Selector7/1 -> adder20/1(In1)
  delayMatch31/1 -> multiplier32/1(In1)
  Selector6/1 -> subtract20/1(In1)
  delayMatch33/1 -> multiplier30/1(In1)
  Selector3/1 -> adder15/1(In1)
  delayMatch35/1 -> multiplier14/1(In1)
  Selector2/1 -> subtract12/1(In1)
  delayMatch37/1 -> multiplier10/1(In1)
  Selector1/1 -> adder11/1(In1)
  Selector/1 -> subtract7/1(In1)
  delayMatch/1 -> multiplier125/1(In1)
  delayMatch1/1 -> multiplier61/1(In1)
  delayMatch2/1 -> adder19/1(In1)
  delayMatch5/1 -> multiplier123/1(In1)
  delayMatch6/1 -> multiplier59/1(In1)
  delayMatch7/1 -> subtract17/1(In1)
  delayMatch10/1 -> multiplier117/1(In1)
  delayMatch12/1 -> multiplier115/1(In1)
  delayMatch14/1 -> multiplier107/1(In1)
  delayMatch16/1 -> multiplier105/1(In1)
  delayMatch18/1 -> multiplier93/1(In1)
  delayMatch20/1 -> multiplier91/1(In1)
  delayMatch22/1 -> multiplier79/1(In1)
  delayMatch24/1 -> multiplier77/1(In1)
  delayMatch26/1 -> multiplier65/1(In1)
  delayMatch28/1 -> multiplier63/1(In1)
  delayMatch30/1 -> multiplier47/1(In1)
  delayMatch32/1 -> multiplier45/1(In1)
  delayMatch34/1 -> multiplier29/1(In1)
  delayMatch36/1 -> multiplier26/1(In1)
  u_dc_link/1 -> concatenate/16, concatenate/15, concatenate/14, concatenate/13, concatenate/12, concatenate/11, concatenate/10, concatenate/9, concatenate/8, concatenate/7, concatenate/6, concatenate/5, concatenate/4, concatenate/3, concatenate/2, concatenate/1
  i_ph_ctrl_alpha/1 -> multiplier15/1(In1)
  i_ph_ctrl_beta/1 -> multiplier11/1(In1)
  omega_el/1 -> multiplier111/2(In2), multiplier97/2(In2), multiplier109/2(In2), multiplier81/2(In2), multiplier83/2(In2), multiplier95/2(In2), multiplier51/2(In2), multiplier67/2(In2), multiplier69/2(In2), multiplier49/2(In2), multiplier33/2(In2), multiplier17/2(In2), multiplier31/2(In2), multiplier13/2(In2), multiplier119/2(In2), multiplier41/2(In2), multiplier43/2(In2), multiplier121/2(In2)
  theta_el/1 -> cos_to_sincos/1(In1)
  Rs/1 -> delayMatch37/1, delayMatch35/1, delayMatch33/1, delayMatch31/1, delayMatch29/1, delayMatch27/1, delayMatch25/1, delayMatch23/1, delayMatch21/1, delayMatch19/1, delayMatch17/1, delayMatch15/1, delayMatch13/1, delayMatch11/1, delayMatch9/1, delayMatch8/1, delayMatch4/1, delayMatch3/1
  reciprocal_Ls/1 -> multiplier124/2(In2), multiplier122/2(In2), multiplier116/2(In2), multiplier114/2(In2), multiplier113/2(In2), multiplier112/2(In2), multiplier106/2(In2), multiplier104/2(In2), multiplier99/2(In2), multiplier98/2(In2), multiplier92/2(In2), multiplier90/2(In2), multiplier85/2(In2), multiplier84/2(In2), multiplier78/2(In2), multiplier76/2(In2), multiplier71/2(In2), multiplier70/2(In2), multiplier64/2(In2), multiplier62/2(In2), multiplier60/2(In2), multiplier58/2(In2), multiplier53/2(In2), multiplier52/2(In2), multiplier46/2(In2), multiplier44/2(In2), multiplier35/2(In2), multiplier34/2(In2), multiplier28/2(In2), multiplier27/2(In2), multiplier25/2(In2), multiplier24/2(In2), multiplier19/2(In2), multiplier18/2(In2), multiplier5/2(In2), multiplier4/2(In2)
  psiPM/1 -> delayMatch36/1, delayMatch34/1, delayMatch32/1, delayMatch30/1, delayMatch28/1, delayMatch26/1, delayMatch24/1, delayMatch22/1, delayMatch20/1, delayMatch18/1, delayMatch16/1, delayMatch14/1, delayMatch12/1, delayMatch10/1, delayMatch6/1, delayMatch5/1, delayMatch1/1, delayMatch/1
  ialpha_ref/1 -> subtract28/1(In1), subtract23/1(In1), subtract15/1(In1), subtract10/1(In1), subtract3/1(In1), subtract5/1(In1), subtract1/1(In1), subtract33/1(In1)
  ibeta_ref/1 -> subtract27/1(In1), subtract22/1(In1), subtract9/1(In1), subtract14/1(In1), subtract4/1(In1), subtract2/1(In1), subtract/1(In1), subtract32/1(In1)
  SampleTime/1 -> multiplier124/1(In1), multiplier122/1(In1), multiplier116/1(In1), multiplier114/1(In1), multiplier113/1(In1), multiplier112/1(In1), multiplier106/1(In1), multiplier104/1(In1), multiplier99/1(In1), multiplier98/1(In1), multiplier92/1(In1), multiplier90/1(In1), multiplier85/1(In1), multiplier84/1(In1), multiplier78/1(In1), multiplier76/1(In1), multiplier71/1(In1), multiplier70/1(In1), multiplier64/1(In1), multiplier62/1(In1), multiplier60/1(In1), multiplier58/1(In1), multiplier53/1(In1), multiplier52/1(In1), multiplier46/1(In1), multiplier44/1(In1), multiplier35/1(In1), multiplier34/1(In1), multiplier28/1(In1), multiplier27/1(In1), multiplier25/1(In1), multiplier24/1(In1), multiplier19/1(In1), multiplier18/1(In1), multiplier5/1(In1), multiplier4/1(In1)
  vk/1 -> Reshape1/1

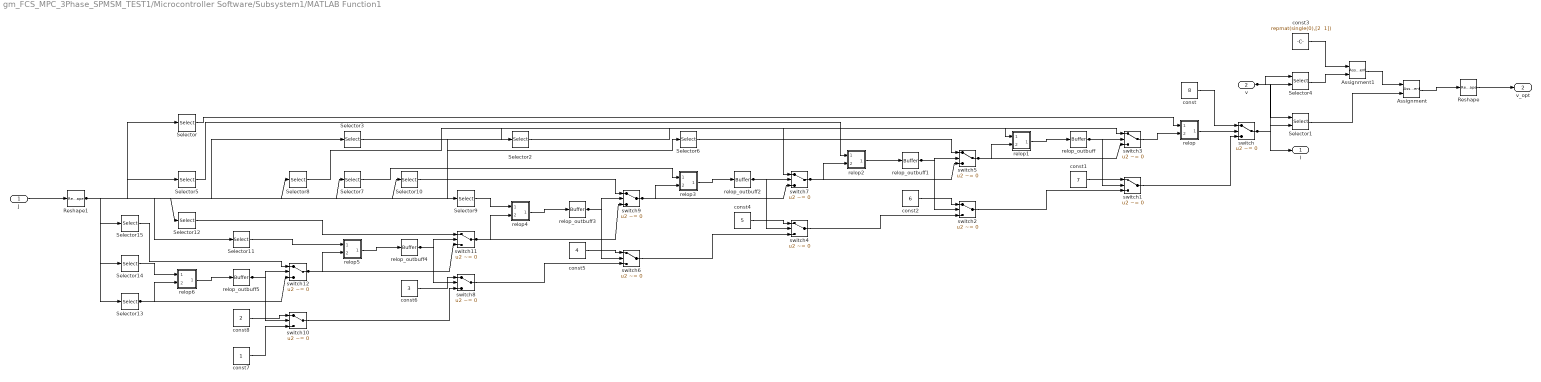
== system gm_FCS_MPC_3Phase_SPMSM_TEST1/Microcontroller Software/Subsystem1/MATLAB Function1 ==
  J : Inport  OutDataTypeStr=single  PortDimensions=[8]  SampleTime=1e-10
  v : Inport  Port=2  OutDataTypeStr=single  PortDimensions=[2,8]  SampleTime=1e-10
  Assignment : Assignment  SampleTime=1e-10  IndexOptions=Index vector (dialog)  Indices=double(2)  OutputSizes=double(0)
  Assignment1 : Assignment  SampleTime=1e-10  IndexOptions=Index vector (dialog)  Indices=double(1)  OutputSizes=double(0)
  Reshape : Reshape
  Reshape1 : Reshape  OutputDimensionality=Column vector (2-D)
  Selector : Selector  SampleTime=1e-10  IndexOptions=Index vector (dialog)  Indices=double(8)  OutputSizes=double(0)
  Selector1 : Selector  NumberOfDimensions=2  SampleTime=1e-10  IndexOptions=Index vector (dialog),Index vector (port)  Indices=double(2),double(-1)  OutputSizes=double(0),double(0)
  Selector10 : Selector  SampleTime=1e-10  IndexOptions=Index vector (dialog)  Indices=double(4)  OutputSizes=double(0)
  Selector11 : Selector  SampleTime=1e-10  IndexOptions=Index vector (dialog)  Indices=double(3)  OutputSizes=double(0)
  Selector12 : Selector  SampleTime=1e-10  IndexOptions=Index vector (dialog)  Indices=double(3)  OutputSizes=double(0)
  Selector13 : Selector  SampleTime=1e-10  IndexOptions=Index vector (dialog)  Indices=double(1)  OutputSizes=double(0)
  Selector14 : Selector  SampleTime=1e-10  IndexOptions=Index vector (dialog)  Indices=double(2)  OutputSizes=double(0)
  Selector15 : Selector  SampleTime=1e-10  IndexOptions=Index vector (dialog)  Indices=double(2)  OutputSizes=double(0)
  Selector2 : Selector  SampleTime=1e-10  IndexOptions=Index vector (dialog)  Indices=double(7)  OutputSizes=double(0)
  Selector3 : Selector  SampleTime=1e-10  IndexOptions=Index vector (dialog)  Indices=double(7)  OutputSizes=double(0)
  Selector4 : Selector  NumberOfDimensions=2  SampleTime=1e-10  IndexOptions=Index vector (dialog),Index vector (port)  Indices=double(1),double(-1)  OutputSizes=double(0),double(0)
  Selector5 : Selector  SampleTime=1e-10  IndexOptions=Index vector (dialog)  Indices=double(6)  OutputSizes=double(0)
  Selector6 : Selector  SampleTime=1e-10  IndexOptions=Index vector (dialog)  Indices=double(6)  OutputSizes=double(0)
  Selector7 : Selector  SampleTime=1e-10  IndexOptions=Index vector (dialog)  Indices=double(5)  OutputSizes=double(0)
  Selector8 : Selector  SampleTime=1e-10  IndexOptions=Index vector (dialog)  Indices=double(5)  OutputSizes=double(0)
  Selector9 : Selector  SampleTime=1e-10  IndexOptions=Index vector (dialog)  Indices=double(4)  OutputSizes=double(0)
  const : Constant  Value=8  VectorParams1D=off  OutDataTypeStr=int32  SampleTime=1e-10
  const1 : Constant  Value=7  VectorParams1D=off  OutDataTypeStr=int32  SampleTime=1e-10
  const2 : Constant  Value=6  VectorParams1D=off  OutDataTypeStr=int32  SampleTime=1e-10
  const3 : Constant  Value="repmat(single(0),[2  1])"  VectorParams1D=off  OutDataTypeStr=single  SampleTime=1e-10
  const4 : Constant  Value=5  VectorParams1D=off  OutDataTypeStr=int32  SampleTime=1e-10
  const5 : Constant  Value=4  VectorParams1D=off  OutDataTypeStr=int32  SampleTime=1e-10
  const6 : Constant  Value=3  VectorParams1D=off  OutDataTypeStr=int32  SampleTime=1e-10
  const7 : Constant  VectorParams1D=off  OutDataTypeStr=int32  SampleTime=1e-10
  const8 : Constant  Value=2  VectorParams1D=off  OutDataTypeStr=int32  SampleTime=1e-10
  relop : Subsystem
      mask Display: disp('NFP\nrelop');
  relop1 : Subsystem
      mask Display: disp('NFP\nrelop');
  relop2 : Subsystem
      mask Display: disp('NFP\nrelop');
  relop3 : Subsystem
      mask Display: disp('NFP\nrelop');
  relop4 : Subsystem
      mask Display: disp('NFP\nrelop');
  relop5 : Subsystem
      mask Display: disp('NFP\nrelop');
  relop6 : Subsystem
      mask Display: disp('NFP\nrelop');
  relop_outbuff{,1..5} (6 alike) : hdlmdlgenlib/Buffer
      settings: SourceProductBaseCode=SL
  switch{,1..2,4,6,8,10} (7 alike) : Switch  Criteria=u2 ~= 0  Threshold=double(0)  OutDataTypeStr=int32  SampleTime=1e-10  SaturateOnIntegerOverflow=off  InputSameDT=off
  switch{3,5,7,9,11..12} (6 alike) : Switch  Criteria=u2 ~= 0  Threshold=double(0)  OutDataTypeStr=single  SampleTime=1e-10  SaturateOnIntegerOverflow=off  InputSameDT=off
  I : Outport  SampleTime=1e-10  VectorParamsAs1DForOutWhenUnconnected=off
  v_opt : Outport  Port=2  SampleTime=1e-10
  wires:
  switch/1 -> Selector4/2, Selector1/2, I/1
  Reshape/1 -> v_opt/1
  const/1 -> switch/1
  Assignment/1 -> Reshape/1
  relop_outbuff/1 -> switch3/2, switch1/2
  const1/1 -> switch1/1
  switch3/1 -> relop/2(In2)
  Selector1/1 -> Assignment/2
  Assignment1/1 -> Assignment/1
  relop_outbuff1/1 -> switch5/2, switch2/2
  const2/1 -> switch2/1
  Reshape1/1 -> Selector15/1, Selector14/1, Selector13/1, Selector12/1, Selector11/1, Selector10/1, Selector9/1, Selector8/1, Selector7/1, Selector6/1, Selector5/1, Selector3/1, Selector2/1, Selector/1
  Selector4/1 -> Assignment1/2
  const3/1 -> Assignment1/1
  relop_outbuff2/1 -> switch7/2, switch4/2
  const4/1 -> switch4/1
  relop_outbuff3/1 -> switch9/2, switch6/2
  const5/1 -> switch6/1
  relop_outbuff4/1 -> switch11/2, switch8/2
  const6/1 -> switch8/1
  const7/1 -> switch10/3
  relop_outbuff5/1 -> switch12/2, switch10/2
  const8/1 -> switch10/1
  Selector14/1 -> relop6/1(In1)
  relop/1(Out1) -> switch/2
  relop1/1(Out1) -> relop_outbuff/1
  relop2/1(Out1) -> relop_outbuff1/1
  relop3/1(Out1) -> relop_outbuff2/1
  relop4/1(Out1) -> relop_outbuff3/1
  relop5/1(Out1) -> relop_outbuff4/1
  relop6/1(Out1) -> relop_outbuff5/1
  Selector15/1 -> switch12/1
  Selector13/1 -> relop6/2(In2), switch12/3
  Selector11/1 -> relop5/1(In1)
  Selector12/1 -> switch11/1
  switch12/1 -> relop5/2(In2), switch11/3
  Selector9/1 -> relop4/1(In1)
  Selector10/1 -> switch9/1
  switch11/1 -> relop4/2(In2), switch9/3
  Selector7/1 -> relop3/1(In1)
  Selector8/1 -> switch7/1
  switch9/1 -> relop3/2(In2), switch7/3
  Selector5/1 -> relop2/1(In1)
  Selector6/1 -> switch5/1
  switch7/1 -> relop2/2(In2), switch5/3
  Selector2/1 -> relop1/1(In1)
  Selector3/1 -> switch3/1
  switch5/1 -> relop1/2(In2), switch3/3
  Selector/1 -> relop/1(In1)
  switch10/1 -> switch8/3
  switch8/1 -> switch6/3
  switch6/1 -> switch4/3
  switch4/1 -> switch2/3
  switch2/1 -> switch1/3
  switch1/1 -> switch/3
  J/1 -> Reshape1/1
  v/1 -> Selector4/1, Selector1/1

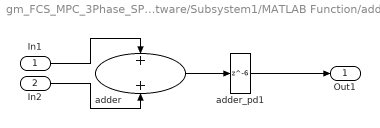
== system gm_FCS_MPC_3Phase_SPMSM_TEST1/Microcontroller Software/Subsystem1/MATLAB Function/adder ==
  In1 : Inport
  In2 : Inport  Port=2
  adder : Sum  OutDataTypeStr=single  SampleTime=1e-10
  adder_pd1 : Delay  DelayLength=6
  Out1 : Outport
  wires:
  In1/1 -> adder/1
  In2/1 -> adder/2
  adder/1 -> adder_pd1/1
  adder_pd1/1 -> Out1/1

== system gm_FCS_MPC_3Phase_SPMSM_TEST1/Microcontroller Software/Subsystem1/MATLAB Function/adder1 ==
  In1 : Inport
  In2 : Inport  Port=2
  adder1 : Sum  OutDataTypeStr=single  SampleTime=1e-10
  adder1_pd1 : Delay  DelayLength=6
  Out1 : Outport
  wires:
  In1/1 -> adder1/1
  In2/1 -> adder1/2
  adder1/1 -> adder1_pd1/1
  adder1_pd1/1 -> Out1/1

== system gm_FCS_MPC_3Phase_SPMSM_TEST1/Microcontroller Software/Subsystem1/MATLAB Function/adder10 ==
  In1 : Inport
  In2 : Inport  Port=2
  adder10 : Sum  OutDataTypeStr=single  SampleTime=1e-10
  adder10_pd1 : Delay  DelayLength=6
  Out1 : Outport
  wires:
  In1/1 -> adder10/1
  In2/1 -> adder10/2
  adder10/1 -> adder10_pd1/1
  adder10_pd1/1 -> Out1/1

== system gm_FCS_MPC_3Phase_SPMSM_TEST1/Microcontroller Software/Subsystem1/MATLAB Function/adder11 ==
  In1 : Inport
  In2 : Inport  Port=2
  adder11 : Sum  OutDataTypeStr=single  SampleTime=1e-10
  adder11_pd1 : Delay  DelayLength=6
  Out1 : Outport
  wires:
  In1/1 -> adder11/1
  In2/1 -> adder11/2
  adder11/1 -> adder11_pd1/1
  adder11_pd1/1 -> Out1/1

== system gm_FCS_MPC_3Phase_SPMSM_TEST1/Microcontroller Software/Subsystem1/MATLAB Function/adder12 ==
  In1 : Inport
  In2 : Inport  Port=2
  adder12 : Sum  OutDataTypeStr=single  SampleTime=1e-10
  adder12_pd1 : Delay  DelayLength=6
  Out1 : Outport
  wires:
  In1/1 -> adder12/1
  In2/1 -> adder12/2
  adder12/1 -> adder12_pd1/1
  adder12_pd1/1 -> Out1/1

== system gm_FCS_MPC_3Phase_SPMSM_TEST1/Microcontroller Software/Subsystem1/MATLAB Function/adder13 ==
  In1 : Inport
  In2 : Inport  Port=2
  adder13 : Sum  OutDataTypeStr=single  SampleTime=1e-10
  adder13_pd1 : Delay  DelayLength=6
  Out1 : Outport
  wires:
  In1/1 -> adder13/1
  In2/1 -> adder13/2
  adder13/1 -> adder13_pd1/1
  adder13_pd1/1 -> Out1/1

== system gm_FCS_MPC_3Phase_SPMSM_TEST1/Microcontroller Software/Subsystem1/MATLAB Function/adder14 ==
  In1 : Inport
  In2 : Inport  Port=2
  adder14 : Sum  OutDataTypeStr=single  SampleTime=1e-10
  adder14_pd1 : Delay  DelayLength=6
  Out1 : Outport
  wires:
  In1/1 -> adder14/1
  In2/1 -> adder14/2
  adder14/1 -> adder14_pd1/1
  adder14_pd1/1 -> Out1/1

== system gm_FCS_MPC_3Phase_SPMSM_TEST1/Microcontroller Software/Subsystem1/MATLAB Function/adder15 ==
  In1 : Inport
  In2 : Inport  Port=2
  adder15 : Sum  OutDataTypeStr=single  SampleTime=1e-10
  adder15_pd1 : Delay  DelayLength=6
  Out1 : Outport
  wires:
  In1/1 -> adder15/1
  In2/1 -> adder15/2
  adder15/1 -> adder15_pd1/1
  adder15_pd1/1 -> Out1/1

== system gm_FCS_MPC_3Phase_SPMSM_TEST1/Microcontroller Software/Subsystem1/MATLAB Function/adder16 ==
  In1 : Inport
  In2 : Inport  Port=2
  adder16 : Sum  OutDataTypeStr=single  SampleTime=1e-10
  adder16_pd1 : Delay  DelayLength=6
  Out1 : Outport
  wires:
  In1/1 -> adder16/1
  In2/1 -> adder16/2
  adder16/1 -> adder16_pd1/1
  adder16_pd1/1 -> Out1/1

== system gm_FCS_MPC_3Phase_SPMSM_TEST1/Microcontroller Software/Subsystem1/MATLAB Function/adder17 ==
  In1 : Inport
  In2 : Inport  Port=2
  adder17 : Sum  OutDataTypeStr=single  SampleTime=1e-10
  adder17_pd1 : Delay  DelayLength=6
  Out1 : Outport
  wires:
  In1/1 -> adder17/1
  In2/1 -> adder17/2
  adder17/1 -> adder17_pd1/1
  adder17_pd1/1 -> Out1/1

== system gm_FCS_MPC_3Phase_SPMSM_TEST1/Microcontroller Software/Subsystem1/MATLAB Function/adder18 ==
  In1 : Inport
  In2 : Inport  Port=2
  adder18 : Sum  OutDataTypeStr=single  SampleTime=1e-10
  adder18_pd1 : Delay  DelayLength=6
  Out1 : Outport
  wires:
  In1/1 -> adder18/1
  In2/1 -> adder18/2
  adder18/1 -> adder18_pd1/1
  adder18_pd1/1 -> Out1/1

== system gm_FCS_MPC_3Phase_SPMSM_TEST1/Microcontroller Software/Subsystem1/MATLAB Function/adder19 ==
  In1 : Inport
  In2 : Inport  Port=2
  adder19 : Sum  OutDataTypeStr=single  SampleTime=1e-10
  adder19_pd1 : Delay  DelayLength=6
  Out1 : Outport
  wires:
  In1/1 -> adder19/1
  In2/1 -> adder19/2
  adder19/1 -> adder19_pd1/1
  adder19_pd1/1 -> Out1/1
